simulink model "ModelNonLinearDig"  (R2014b)
settings: Solver=ode23  StartTime=0.0  StopTime=15  FixedStep=0.001  RelTol=1e-3
InitFcn:
  | InitModel;
values from neighbouring files (symbols this model uses):
  C1_dig = c2d(tf(C1_dig),0.0001,'tustin')    [InitModel.m]
  Kpwm = 1/8    (= 0.125)    [InitModel.m]
  R1 = 1.8e3    (= 1800)    [InitModel.m]    (also in SystemModel.m; SystemModel_marco.m)
  R4 = 47e3    (= 47000)    [InitModel.m]    (also in SystemModel.m; SystemModel_marco.m)
  rad2rpm = 60/(2*pi)    (= 9.54929658551)    [InitModel.m]    (also in SystemModel.m)
  Rs = 0.1    [InitModel.m]    (also in SystemModel.m; SystemModel_marco.m)
  sp = misureB.shaftSpeed    [betacalcs.m]    (also in computeFrictionParams.m = misureB.tach * 1/tach.gain; validation.m = 1)
  tau = misureB.frictionTorque    [betacalcs.m]    (also in computeFrictionParams.m)
  Vdc = 30    [InitModel.m]    (also in SystemModel.m; SystemModel_marco.m)
undefined symbols (not defined in the file or in its folder): motor, sigbuilder_block, tach
libraries: cstblocks x4, simulink_extras x2, simulink x1
settings Model: Creator=Edoardo  LastModifiedBy=Edoardo
settings SolverCC: ZeroCrossAlgorithm=Adaptive  PositivePriorityOrder=on
settings DataIOCC: SaveOutput=off  SaveTime=off

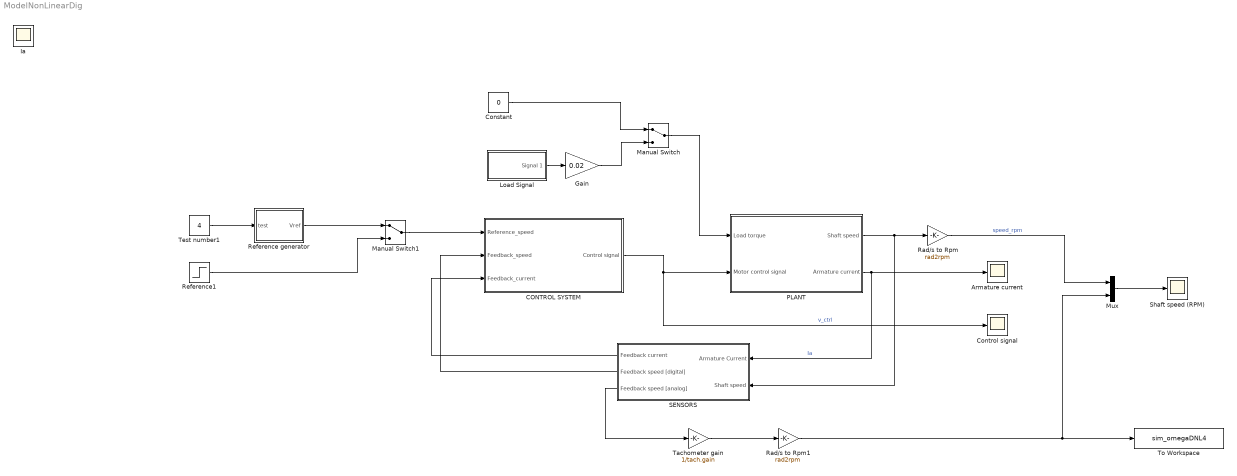
== system ModelNonLinearDig ==
  "Armature current " : Scope
      settings: YMin=0  YMax=7  SaveName=ScopeData3
  CONTROL SYSTEM : Subsystem
  Constant : Constant  Value=0
  Control signal : Scope
      settings: YMin=-0.2  YMax=1.4  SaveName=ScopeData5
  Gain : Gain  Gain=0.02
  Load Signal : Subsystem  Tag=STV Subsys  LoadFcn=sigbuilder_block('load');  StartFcn=sigbuilder_block('start');  StopFcn=sigbuilder_block('stop');  ClipboardFcn=sigbuilder_block('clipboard');  mask(Sigbuilder block){}
      mask help: Simulink:masks:SigbuilderBlock_MD
      mask init:
      | if ~strcmp(get_param(bdroot(gcbh),'SimulationStatus'),'stopped') tuvar = sigbuilder_block('maskInit'); end
      settings: CopyFcn=sigbuilder_block('copy');  DeleteFcn=sigbuilder_block('delete');  ModelCloseFcn=sigbuilder_block('modelClose');  PreSaveFcn=sigbuilder_block('preSave');  PauseFcn=sigbuilder_block('pause');  ContinueFcn=sigbuilder_block('continue');  NameChangeFcn=sigbuilder_block('namechange');  OpenFcn=sigbuilder_block('open',[437.6 199.2 550.4 400 ]);  CloseFcn=sigbuilder_block('close');
      mask Display: plot(0, 0, 100, 100,[2, 2, 32, 32, 2], [68, 8, 8, 68, 68],[32, 2], [38, 38], [32, 19, 2],[53, 60, 44], [32, 17, 17, 2],[16, 16, 31, 31]);txt = getActiveGroup(gcbh);text(2, 100, txt,'verticalAlignment', 'top');
  Manual Switch : ManualSwitch
  Manual Switch1 : ManualSwitch
  Mux : Mux  Inputs=2
  PLANT : Subsystem
  Rad/s to Rpm : Gain  Gain=rad2rpm
  Rad/s to Rpm1 : Gain  Gain=rad2rpm
  Reference generator : Subsystem
  Reference1 : Step  Time=0  SampleTime=0
  SENSORS : Subsystem
  Shaft speed (RPM) : Scope
      settings: ShowLegends=on  TimeRange=1  YMin=-1
  Tachometer gain : Gain  Gain=1/tach.gain
  Test number1 : Constant  Value=4
  To Workspace : ToWorkspace  VariableName=sim_omegaDNL4  SaveFormat=Timeseries  SampleTime=-1
      settings: Save2DSignal=2-D array (concatenate along first dimension)
  Ia : Scope
  wires:
  Rad/s to Rpm/1 -> Mux/1  "speed_rpm"
  PLANT/1(Shaft speed) -> SENSORS/2(Shaft speed), Rad/s to Rpm/1
  CONTROL SYSTEM/1(Control signal) -> Control signal/1, PLANT/2(Motor control signal)  "v_ctrl"
  PLANT/2(Armature current) -> SENSORS/1(Armature Current), "Armature current "/1  "Ia"
  SENSORS/1(Feedback current) -> CONTROL SYSTEM/3(Feedback_current)
  Manual Switch/1 -> PLANT/1(Load torque)
  Constant/1 -> Manual Switch/1
  Load Signal/1(Signal 1) -> Gain/1
  Gain/1 -> Manual Switch/2
  Manual Switch1/1 -> CONTROL SYSTEM/1(Reference_speed)
  SENSORS/2("Feedback speed [digital] ") -> CONTROL SYSTEM/2(Feedback_speed)
  Tachometer gain/1 -> Rad/s to Rpm1/1
  Rad/s to Rpm1/1 -> Mux/2, To Workspace/1
  Mux/1 -> Shaft speed (RPM)/1
  Reference1/1 -> Manual Switch1/2
  Reference generator/1(Vref) -> Manual Switch1/1
  Test number1/1 -> Reference generator/1(test)
  SENSORS/3(Feedback speed [analog]) -> Tachometer gain/1

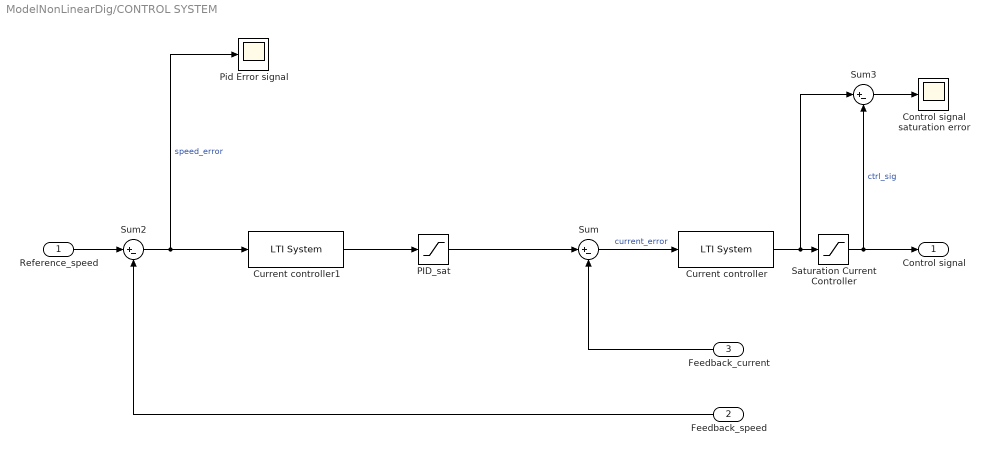
== system ModelNonLinearDig/CONTROL SYSTEM ==
  Reference_speed : Inport
  Feedback_speed : Inport  Port=2
  Feedback_current : Inport  Port=3
  Control signal saturation error : Scope
      settings: YMin=-1  YMax=1  SaveName=ScopeData4  Decimation=10
  Current controller : cstblocks/LTI System  sys=-C1_dig  IC=[]
  Current controller1 : cstblocks/LTI System  sys=C2_dig  IC=[]
  PID_sat : Saturate  UpperLimit=2  LowerLimit=-2
  Pid Error signal : Scope
      settings: SaveName=ScopeData10  Decimation=20
  Saturation Current Controller : Saturate  UpperLimit=10  LowerLimit=-10
  Sum : Sum  Inputs=|+-
  Sum2 : Sum  Inputs=|+-
  Sum3 : Sum  Inputs=|+-
  Control signal : Outport
  wires:
  Current controller/1 -> Sum3/1, Saturation Current Controller/1
  Sum/1 -> Current controller/1  "current_error"
  Feedback_current/1 -> Sum/2
  Saturation Current Controller/1 -> Control signal/1, Sum3/2  "ctrl_sig"
  Reference_speed/1 -> Sum2/1
  Feedback_speed/1 -> Sum2/2
  Sum2/1 -> Current controller1/1, Pid Error signal/1  "speed_error"
  Sum3/1 -> Control signal saturation error/1
  Current controller1/1 -> PID_sat/1
  PID_sat/1 -> Sum/1

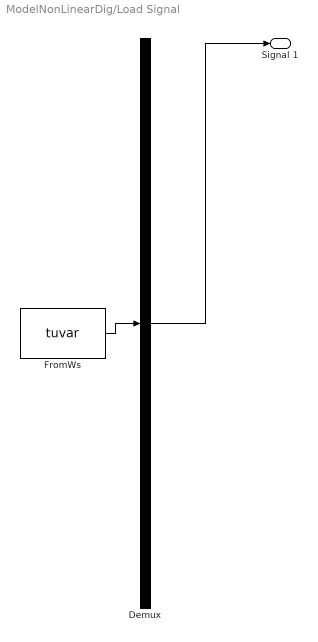
== system ModelNonLinearDig/Load Signal ==
  Demux : Demux  Tag=STV Demux  Outputs=1
  FromWs : FromWorkspace  Tag=STV FromWs  VariableName=tuvar  SampleTime=0
      SigBuilderData=|
      | common.afterFinalStr = 'Extrapolate'
      | common.sampleTime = 0
      | dataSet.timeRange = [0 10]
      | dataSet.name = 'Group 1'
      | sbobj.Groups.Name = 'Group 1'
      | sbobj.Groups.Signals.Name = 'Signal 1'
      | sbobj.Groups.Signals.XData = [0 1.8 2 6 6 10]
      | sbobj.Groups.Signals.YData = [0 0 1 1 0 0]
  Signal 1 : Outport  Tag=STV Outport
  wires:
  Demux/1 -> Signal 1/1
  FromWs/1 -> Demux/1

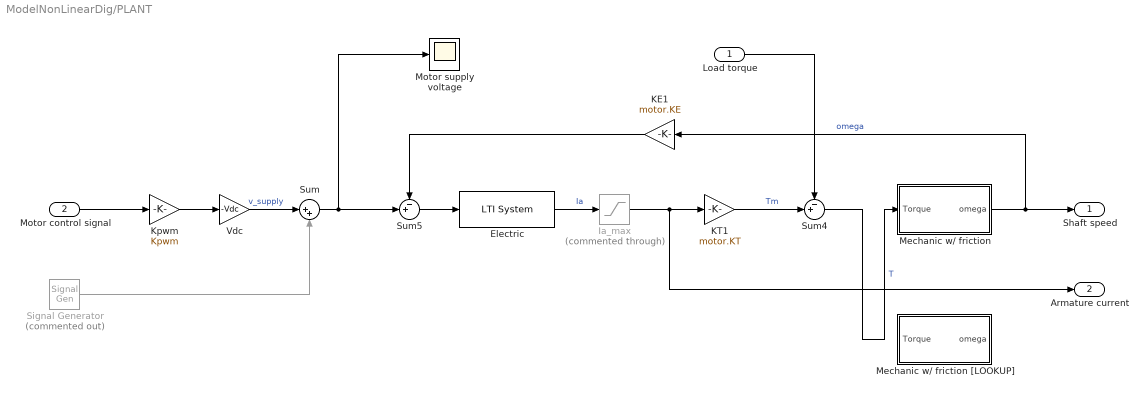
== system ModelNonLinearDig/PLANT ==
  Load torque : Inport
  Motor control signal : Inport  Port=2
  Electric : cstblocks/LTI System  sys=G1  IC=[]
  Ia_max : Saturate  Commented=through  UpperLimit=motor.Ia_max  LowerLimit=-motor.Ia_max
  KE1 : Gain  Gain=motor.KE
  KT1 : Gain  Gain=motor.KT
  Kpwm : Gain  Gain=Kpwm
  Mechanic w/ friction : Subsystem
  Mechanic w/ friction [LOOKUP] : Subsystem
  Motor supply voltage : Scope
      settings: SaveName=ScopeData2
  Signal Generator : SignalGenerator  Commented=on  WaveForm=square  Amplitude=0.03  Frequency=23e3
  Sum : Sum  Inputs=|++
  Sum4 : Sum  Inputs=-+|
  Sum5 : Sum  Inputs=-+|
  Vdc : Gain  Gain=-Vdc
  Shaft speed : Outport
  Armature current : Outport  Port=2
  wires:
  Electric/1 -> Ia_max/1  "Ia"
  Motor control signal/1 -> Kpwm/1
  Sum5/1 -> Electric/1
  KE1/1 -> Sum5/1
  Ia_max/1 -> KT1/1, Armature current/1
  Load torque/1 -> Sum4/1
  KT1/1 -> Sum4/2  "Tm"
  Vdc/1 -> Sum/1  "v_supply"
  Signal Generator/1 -> Sum/2
  Sum/1 -> Motor supply voltage/1, Sum5/2
  Kpwm/1 -> Vdc/1
  Sum4/1 -> Mechanic w/ friction/1(Torque)  "T"
  Mechanic w/ friction/1(omega) -> KE1/1, Shaft speed/1  "omega"

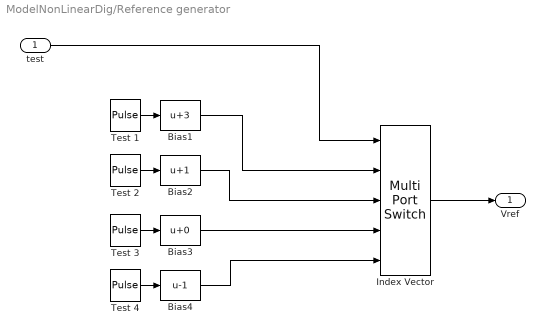
== system ModelNonLinearDig/Reference generator ==
  test : Inport
  Bias1 : Bias  Bias=3
  Bias2 : Bias  Bias=1
  Bias3 : Bias
  Bias4 : Bias  Bias=-1
  Index Vector : MultiPortSwitch  Inputs=4
  Test 1 : DiscretePulseGenerator  PulseType=Time based  Amplitude=2  Period=5  PulseWidth=50  PhaseDelay=1
  Test 2 : DiscretePulseGenerator  PulseType=Time based  Amplitude=6  Period=5  PulseWidth=50  PhaseDelay=1
  Test 3 : DiscretePulseGenerator  PulseType=Time based  Amplitude=8  Period=5  PulseWidth=50  PhaseDelay=1
  Test 4 : DiscretePulseGenerator  PulseType=Time based  Amplitude=2  Period=5  PulseWidth=50  PhaseDelay=1
  Vref : Outport
  wires:
  Test 4/1 -> Bias4/1
  Bias4/1 -> Index Vector/5
  Test 1/1 -> Bias1/1
  Test 2/1 -> Bias2/1
  Bias2/1 -> Index Vector/3
  test/1 -> Index Vector/1
  Bias3/1 -> Index Vector/4
  Test 3/1 -> Bias3/1
  Bias1/1 -> Index Vector/2
  Index Vector/1 -> Vref/1

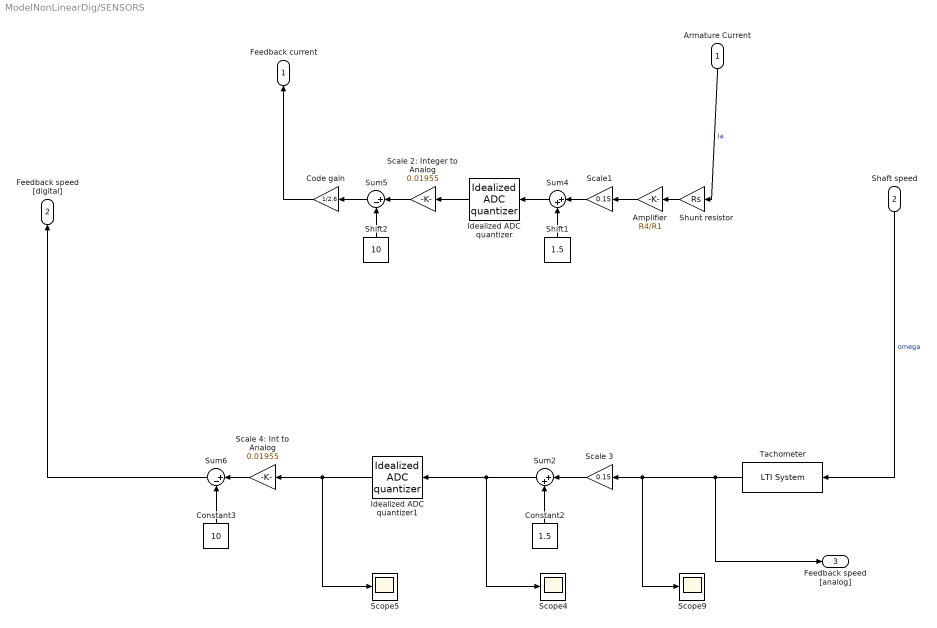
== system ModelNonLinearDig/SENSORS ==
  Armature Current : Inport
  Shaft speed : Inport  Port=2
  " Amplifier " : Gain  Gain=R4/R1
  " Code gain" : Gain  Gain=1/2.6
  " Scale 3" : Gain  Gain=0.15
  " Scale 4: Int to Analog" : Gain  Gain=0.01955
  " Scale1" : Gain  Gain=0.15
  " Shunt resistor" : Gain  Gain=Rs
  Constant2 : Constant  Value=1.5
  Constant3 : Constant  Value=10
  Idealized ADC quantizer : simulink_extras/Additional Discrete/Idealized ADC quantizer  NumberOfConverterBits=10  Vmin=0  Vmax=3  OutputDataType=uint16  OutputNegativeValues=on
  Idealized ADC quantizer1 : simulink_extras/Additional Discrete/Idealized ADC quantizer  NumberOfConverterBits=10  Vmin=0  Vmax=3  OutputDataType=uint16  OutputNegativeValues=on
  Scale 2: Integer to Analog : Gain  Gain=0.01955
  Scope4 : Scope
      settings: YMin=-3.95  YMax=-3.75  SaveName=ScopeData6  Decimation=10
  Scope5 : Scope
      settings: YMin=500  YMax=1100  SaveName=ScopeData7  Decimation=10
  Scope9 : Scope
      settings: YMax=35  SaveName=ScopeData8  Decimation=10
  Shift1 : Constant  Value=1.5
  Shift2 : Constant  Value=10
  Sum2 : Sum  Inputs=|++
  Sum4 : Sum  Inputs=|++
  Sum5 : Sum  Inputs=|+-
  Sum6 : Sum  Inputs=|+-
  Tachometer : cstblocks/LTI System  sys=H2  IC=[]
  Feedback current : Outport
  "Feedback speed [digital] " : Outport  Port=2
  Feedback speed [analog] : Outport  Port=3
  wires:
  Armature Current/1 -> " Shunt resistor"/1  "Ia"
  " Shunt resistor"/1 -> " Amplifier "/1
  " Amplifier "/1 -> " Scale1"/1
  " Scale1"/1 -> Sum4/1
  Shift1/1 -> Sum4/2
  Sum4/1 -> Idealized ADC quantizer/1
  Idealized ADC quantizer/1 -> Scale 2: Integer to Analog/1
  Scale 2: Integer to Analog/1 -> Sum5/1
  Shift2/1 -> Sum5/2
  Sum5/1 -> " Code gain"/1
  " Code gain"/1 -> Feedback current/1
  Shaft speed/1 -> Tachometer/1  "omega"
  Constant2/1 -> Sum2/2
  " Scale 3"/1 -> Sum2/1
  Sum2/1 -> Scope4/1, Idealized ADC quantizer1/1
  Idealized ADC quantizer1/1 -> Scope5/1, " Scale 4: Int to Analog"/1
  " Scale 4: Int to Analog"/1 -> Sum6/1
  Constant3/1 -> Sum6/2
  Tachometer/1 -> Feedback speed [analog]/1, Scope9/1, " Scale 3"/1
  Sum6/1 -> "Feedback speed [digital] "/1

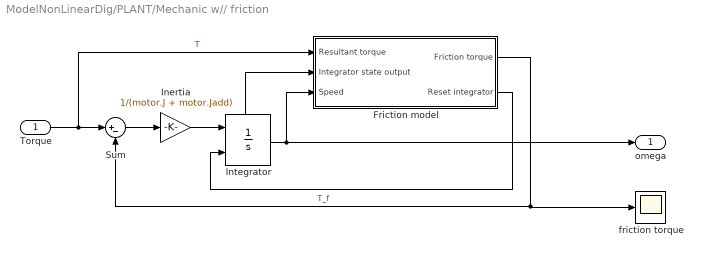
== system ModelNonLinearDig/PLANT/Mechanic w// friction ==
  Torque : Inport
  Friction model : Subsystem
  Inertia : Gain  Gain=1/(motor.J + motor.Jadd)
  Integrator : Integrator  ExternalReset=rising  ShowStatePort=on
  Sum : Sum  Inputs=|+-
  friction torque : Scope
      settings: YMin=0.0075  YMax=0.0125  SaveName=ScopeData9
  omega : Outport
  wires:
  Torque/1 -> Sum/1, Friction model/1(Resultant torque)  "T"
  Inertia/1 -> Integrator/1
  Friction model/1(Friction torque) -> friction torque/1, Sum/2  "T_f"
  Integrator/State -> Friction model/2(Integrator state output)
  Integrator/1 -> omega/1, Friction model/3(Speed)
  Sum/1 -> Inertia/1
  Friction model/2(Reset integrator) -> Integrator/2

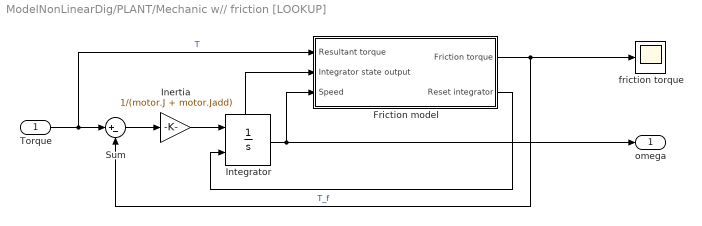
== system ModelNonLinearDig/PLANT/Mechanic w// friction [LOOKUP] ==
  Torque : Inport
  Friction model : Subsystem
  Inertia : Gain  Gain=1/(motor.J + motor.Jadd)
  Integrator : Integrator  ExternalReset=rising  ShowStatePort=on
  Sum : Sum  Inputs=|+-
  friction torque : Scope
      settings: YMin=0.0075  YMax=0.0125  SaveName=ScopeData9
  omega : Outport
  wires:
  Friction model/2(Reset integrator) -> Integrator/2
  Sum/1 -> Inertia/1
  Integrator/1 -> Friction model/3(Speed), omega/1
  Integrator/State -> Friction model/2(Integrator state output)
  Friction model/1(Friction torque) -> Sum/2, friction torque/1  "T_f"
  Inertia/1 -> Integrator/1
  Torque/1 -> Friction model/1(Resultant torque), Sum/1  "T"

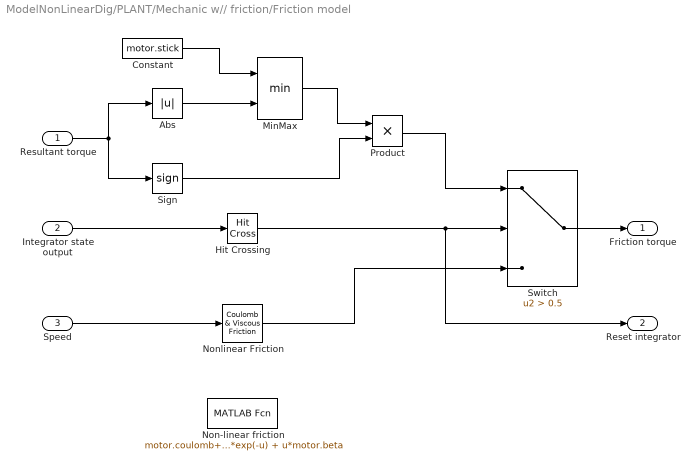
== system ModelNonLinearDig/PLANT/Mechanic w// friction/Friction model ==
  Resultant torque : Inport
  Integrator state output : Inport  Port=2
  Speed : Inport  Port=3
  Abs : Abs
  Constant : Constant  Value=motor.stick
  Hit Crossing : HitCross
  MinMax : MinMax  Inputs=2
  Non-linear friction : MATLABFcn  MATLABFcn=motor.coulomb+(motor.stick - motor.coulomb)*exp(-u) + u*motor.beta
  Nonlinear Friction : simulink/Discontinuities/Coulomb & Viscous Friction  offset=motor.coulomb  gain=motor.beta
  Product : Product
  Sign : Signum
  Switch : Switch  Criteria=u2 > Threshold  Threshold=0.5
  Friction torque : Outport
  Reset integrator : Outport  Port=2
  wires:
  MinMax/1 -> Product/1
  Constant/1 -> MinMax/1
  Sign/1 -> Product/2
  Abs/1 -> MinMax/2
  Product/1 -> Switch/1
  Integrator state output/1 -> Hit Crossing/1
  Switch/1 -> Friction torque/1
  Resultant torque/1 -> Sign/1, Abs/1
  Hit Crossing/1 -> Reset integrator/1, Switch/2
  Speed/1 -> Nonlinear Friction/1
  Nonlinear Friction/1 -> Switch/3

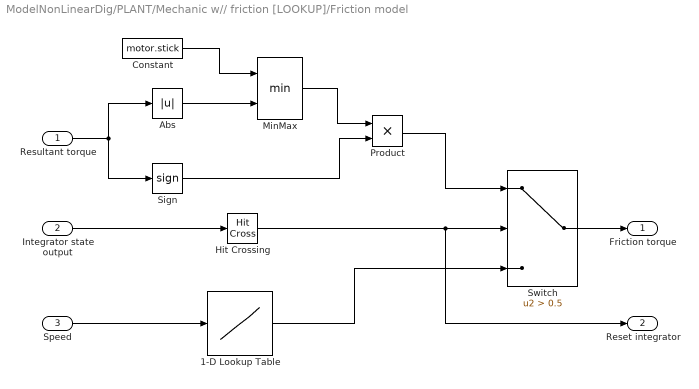
== system ModelNonLinearDig/PLANT/Mechanic w// friction [LOOKUP]/Friction model ==
  Resultant torque : Inport
  Integrator state output : Inport  Port=2
  Speed : Inport  Port=3
  1-D Lookup Table : Lookup_n-D  NumberOfTableDimensions=1  BreakpointsForDimension1=sp  Table=tau  InternalRulePriority=Speed  RndMeth=Simplest  InputSameDT=on
  Abs : Abs
  Constant : Constant  Value=motor.stick
  Hit Crossing : HitCross
  MinMax : MinMax  Inputs=2
  Product : Product
  Sign : Signum
  Switch : Switch  Criteria=u2 > Threshold  Threshold=0.5
  Friction torque : Outport
  Reset integrator : Outport  Port=2
  wires:
  1-D Lookup Table/1 -> Switch/3
  Speed/1 -> 1-D Lookup Table/1
  Hit Crossing/1 -> Switch/2, Reset integrator/1
  Resultant torque/1 -> Abs/1, Sign/1
  Switch/1 -> Friction torque/1
  Integrator state output/1 -> Hit Crossing/1
  Product/1 -> Switch/1
  Abs/1 -> MinMax/2
  Sign/1 -> Product/2
  Constant/1 -> MinMax/1
  MinMax/1 -> Product/1
